simulink library "wt_blockset_v3"  (Simulink 6.0)
settings: Solver=ode45  SolverMode=SingleTasking  StartTime=0.0  StopTime=10.0  RelTol=1e-3
undefined symbols (not defined in the file): f1, get, j, Kmode, Type, u0
libraries: simulink_extras x12, simulink3 x5, simulink x4, dspinverses x1, dspmtrx3 x1, dspsnks4 x1
(part 3 of 7)

== system wt_blockset_v3/Mechanical Components/Wind Model SB-1 ==
  omg_wt : Inport  Port=1  LatchInput=off
  0 Harmonic Filter : TransferFcn  Numerator=[0 4.7869*d 0.9904]  Denominator=[7.6823*d^2 7.3518*d 1]
  3 Harmonic : Sum  SaturateOnIntegerOverflow=on  InputSameDT=on
  3 Harmonic Filter_1 : TransferFcn  Numerator=[0 0.2766*d 0.0307]  Denominator=[0.3691*d^2 1.7722*d 1]
  3 Harmonic Filter_2 : TransferFcn  Numerator=[0 0.2766*d 0.0307]  Denominator=[0.3691*d^2 1.7722*d 1]
  Clock : Clock
  Constant1 : Constant  Value=v_mean
  Gain : Gain  Gain=2*pi/60  SaturateOnIntegerOverflow=on
  Kaimal_Filter_1 : Subsystem
  Kaimal_Filter_2 : Subsystem
  Kaimal_Filter_3 : Subsystem
  Mux : Mux  Inputs=2
  Product : Product  SaturateOnIntegerOverflow=on  InputSameDT=on
  Product1 : Product  SaturateOnIntegerOverflow=on  InputSameDT=on
  Sum : Sum  SaturateOnIntegerOverflow=on  InputSameDT=on
  Sum2 : Sum  SaturateOnIntegerOverflow=on  InputSameDT=on
  Unit Delay : UnitDelay  SampleTime=T_sample
  Unit Delay1 : UnitDelay  SampleTime=T_sample
  White Noise_1 : Subsystem  mask(Continuous White Noise.){Cov=[1], Ts=T_sample, seed=[random(1)]}
      mask prompts: Cov "Noise Power:"; Ts "Sample Time:"
      mask help:
      | White noise for continuous (s-domain) systems.
      | Band-limited using zero-order-hold.
      mask init:
      | r = rand(1,12); r2 = [r(1),r;r,r(12)]; t =[1:13;1:13];
      mask Help: Implemented using white noise into Zero-Order Hold block. The seed and power can be vectors of the same length to produce a vector of white noise sources. For faster simulation, set sample time to the highest value possible but in accordance with the fastest dynamics of system.
      mask Display: plot(t(:),r2(:))
  White Noise_2 : Subsystem  mask(Continuous White Noise.){@1=[1], @2=T_sample, @3=[random(2)]}
      mask prompts: @1 "Noise Power:"; @2 "Sample Time:"; @3 "Seed"
      mask help:
      | White noise for continuous (s-domain) systems.
      | Band-limited using zero-order-hold.
      mask init:
      | Cov = @1; Ts = @2; seed = @3; r = rand(1,12); r2 = [r(1),r;r,r(12)]; t =[1:13;1:13];
      mask Help: Implemented using white noise into Zero-Order Hold block. The seed and power can be vectors of the same length to produce a vector of white noise sources. For faster simulation, set sample time to the highest value possible but in accordance with the fastest dynamics of system.
      mask Display: plot(t(:),r2(:))
  White Noise_3 : Subsystem  mask(Continuous White Noise.){@1=[1], @2=T_sample, @3=[random(3)]}
      mask prompts: @1 "Noise Power:"; @2 "Sample Time:"; @3 "Seed"
      mask help:
      | White noise for continuous (s-domain) systems.
      | Band-limited using zero-order-hold.
      mask init:
      | Cov = @1; Ts = @2; seed = @3; r = rand(1,12); r2 = [r(1),r;r,r(12)]; t =[1:13;1:13];
      mask Help: Implemented using white noise into Zero-Order Hold block. The seed and power can be vectors of the same length to produce a vector of white noise sources. For faster simulation, set sample time to the highest value possible but in accordance with the fastest dynamics of system.
      mask Display: plot(t(:),r2(:))
  cos fun : Fcn  Expr=sqrt(2)*cos(3*u[1]*u[2])
  sin fun : Fcn  Expr=sqrt(2)*sin(3*u[1]*u[2])
  wind : Outport  InitialOutput=[u0]
  wires:
  Kaimal_Filter_2/1(out_1) -> 3 Harmonic Filter_1/1
  Kaimal_Filter_3/1(out_1) -> 3 Harmonic Filter_2/1
  cos fun/1 -> Unit Delay/1
  sin fun/1 -> Unit Delay1/1
  Product/1 -> 3 Harmonic/1
  Product1/1 -> 3 Harmonic/2
  3 Harmonic Filter_2/1 -> Product1/2
  3 Harmonic/1 -> Sum/2
  0 Harmonic Filter/1 -> Sum2/2
  Sum2/1 -> Sum/1
  Constant1/1 -> Sum2/1
  Sum/1 -> wind/1
  Kaimal_Filter_1/1(out_1) -> 0 Harmonic Filter/1
  White Noise_1/1(Out_1) -> Kaimal_Filter_1/1(in_1)
  White Noise_2/1(Out_1) -> Kaimal_Filter_2/1(in_1)
  White Noise_3/1(Out_1) -> Kaimal_Filter_3/1(in_1)
  3 Harmonic Filter_1/1 -> Product/1
  Mux/1 -> cos fun/1, sin fun/1
  omg_wt/1 -> Gain/1
  Gain/1 -> Mux/1
  Unit Delay/1 -> Product/2
  Unit Delay1/1 -> Product1/1
  Clock/1 -> Mux/2

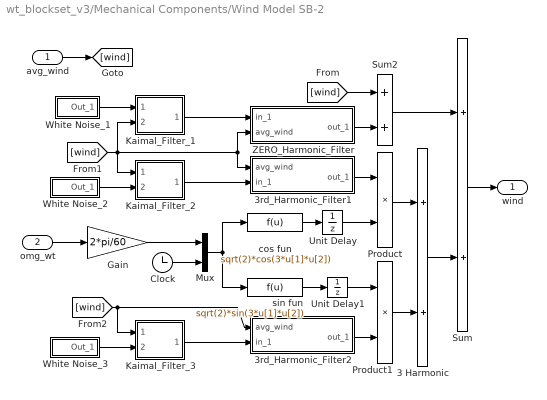
== system wt_blockset_v3/Mechanical Components/Wind Model SB-2 ==
  avg_wind : Inport  Port=1  LatchInput=off
  omg_wt : Inport  Port=2  LatchInput=off
  3 Harmonic : Sum  SaturateOnIntegerOverflow=on  InputSameDT=on
  3rd_Harmonic_Filter1 : Subsystem
  3rd_Harmonic_Filter2 : Subsystem
  Clock : Clock
  Gain : Gain  Gain=2*pi/60  SaturateOnIntegerOverflow=on
  Kaimal_Filter_1 : Subsystem
  Kaimal_Filter_2 : Subsystem
  Kaimal_Filter_3 : Subsystem
  Mux : Mux  Inputs=2
  Product : Product  SaturateOnIntegerOverflow=on  InputSameDT=on
  Product1 : Product  SaturateOnIntegerOverflow=on  InputSameDT=on
  Sum : Sum  SaturateOnIntegerOverflow=on  InputSameDT=on
  Sum2 : Sum  SaturateOnIntegerOverflow=on  InputSameDT=on
  Unit Delay : UnitDelay  SampleTime=T_sample
  Unit Delay1 : UnitDelay  SampleTime=T_sample
  White Noise_1 : Subsystem  mask(Continuous White Noise.){Cov=[1], Ts=T_sample, seed=[random(1)]}
      mask prompts: Cov "Noise Power:"; Ts "Sample Time:"
      mask help:
      | White noise for continuous (s-domain) systems.
      | Band-limited using zero-order-hold.
      mask init:
      | r = rand(1,12); r2 = [r(1),r;r,r(12)]; t =[1:13;1:13];
      mask Help: Implemented using white noise into Zero-Order Hold block. The seed and power can be vectors of the same length to produce a vector of white noise sources. For faster simulation, set sample time to the highest value possible but in accordance with the fastest dynamics of system.
      mask Display: plot(t(:),r2(:))
  White Noise_2 : Subsystem  mask(Continuous White Noise.){@1=[1], @2=T_sample, @3=[random(2)]}
      mask prompts: @1 "Noise Power:"; @2 "Sample Time:"; @3 "Seed"
      mask help:
      | White noise for continuous (s-domain) systems.
      | Band-limited using zero-order-hold.
      mask init:
      | Cov = @1; Ts = @2; seed = @3; r = rand(1,12); r2 = [r(1),r;r,r(12)]; t =[1:13;1:13];
      mask Help: Implemented using white noise into Zero-Order Hold block. The seed and power can be vectors of the same length to produce a vector of white noise sources. For faster simulation, set sample time to the highest value possible but in accordance with the fastest dynamics of system.
      mask Display: plot(t(:),r2(:))
  White Noise_3 : Subsystem  mask(Continuous White Noise.){@1=[1], @2=T_sample, @3=[random(3)]}
      mask prompts: @1 "Noise Power:"; @2 "Sample Time:"; @3 "Seed"
      mask help:
      | White noise for continuous (s-domain) systems.
      | Band-limited using zero-order-hold.
      mask init:
      | Cov = @1; Ts = @2; seed = @3; r = rand(1,12); r2 = [r(1),r;r,r(12)]; t =[1:13;1:13];
      mask Help: Implemented using white noise into Zero-Order Hold block. The seed and power can be vectors of the same length to produce a vector of white noise sources. For faster simulation, set sample time to the highest value possible but in accordance with the fastest dynamics of system.
      mask Display: plot(t(:),r2(:))
  ZERO_Harmonic_Filter : Subsystem
  cos fun : Fcn  Expr=sqrt(2)*cos(3*u[1]*u[2])
  sin fun : Fcn  Expr=sqrt(2)*sin(3*u[1]*u[2])
  wind : Outport  InitialOutput=[u0]
  wires:
  Clock/1 -> Mux/2
  Unit Delay1/1 -> Product1/1
  Unit Delay/1 -> Product/2
  Gain/1 -> Mux/1
  omg_wt/1 -> Gain/1
  Mux/1 -> sin fun/1, cos fun/1
  3rd_Harmonic_Filter1/1(out_1) -> Product/1
  White Noise_3/1(Out_1) -> Kaimal_Filter_3/2(in_1)
  White Noise_1/1(Out_1) -> Kaimal_Filter_1/1(in_1)
  Sum/1 -> wind/1
  [wind] -> Sum2/1
  Sum2/1 -> Sum/1
  ZERO_Harmonic_Filter/1(out_1) -> Sum2/2
  3 Harmonic/1 -> Sum/2
  3rd_Harmonic_Filter2/1(out_1) -> Product1/2
  Product1/1 -> 3 Harmonic/2
  Product/1 -> 3 Harmonic/1
  sin fun/1 -> Unit Delay1/1
  cos fun/1 -> Unit Delay/1
  Kaimal_Filter_1/1(out_1) -> ZERO_Harmonic_Filter/1(in_1)
  Kaimal_Filter_2/1(out_1) -> 3rd_Harmonic_Filter1/2(in_1)
  White Noise_2/1(Out_1) -> Kaimal_Filter_2/2(in_1)
  avg_wind/1 -> [wind]
  [wind] -> Kaimal_Filter_1/2(avg_wind), Kaimal_Filter_2/1(avg_wind), ZERO_Harmonic_Filter/2(avg_wind), 3rd_Harmonic_Filter1/1(avg_wind)
  [wind] -> Kaimal_Filter_3/1(avg_wind), 3rd_Harmonic_Filter2/1(avg_wind)
  Kaimal_Filter_3/1(out_1) -> 3rd_Harmonic_Filter2/2(in_1)

== system wt_blockset_v3/Mechanical Components/Wind Model ZA-1 ==
  omg_wt : Inport  Port=1  LatchInput=off
  0 Harmonic Filter : TransferFcn  Numerator=[0 4.7869*d 0.9904]  Denominator=[7.6823*d^2 7.3518*d 1]
  3 Harmonic : Sum  SaturateOnIntegerOverflow=on  InputSameDT=on
  3 Harmonic Filter_1 : TransferFcn  Numerator=[0 0.2766*d 0.0307]  Denominator=[0.3691*d^2 1.7722*d 1]
  3 Harmonic Filter_2 : TransferFcn  Numerator=[0 0.2766*d 0.0307]  Denominator=[0.3691*d^2 1.7722*d 1]
  Band Limited White Noise : Subsystem  mask(Band Limited White Noise Generator){noise=1, seed=256, T_sample=0.05}
      mask prompts: noise "noise power"; T_sample "sample time [sec]"
      mask help: Implements a Band Limited White Noise Generator using the Marsaglia's ziggurat method.
      mask Display: disp('White Noise')
  Band Limited White Noise1 : Subsystem  mask(Band Limited White Noise Generator){noise=1, seed=894, T_sample=0.05}
      mask prompts: noise "noise power"; T_sample "sample time [sec]"
      mask help: Implements a Band Limited White Noise Generator using the Marsaglia's ziggurat method.
      mask Display: disp('White Noise')
  Band Limited White Noise2 : Subsystem  mask(Band Limited White Noise Generator){noise=1, seed=31, T_sample=0.05}
      mask prompts: noise "noise power"; T_sample "sample time [sec]"
      mask help: Implements a Band Limited White Noise Generator using the Marsaglia's ziggurat method.
      mask Display: disp('White Noise')
  Clock : Clock
  Constant1 : Constant  Value=v_mean
  Gain : Gain  Gain=2*pi/60  SaturateOnIntegerOverflow=on
  Kaimal_Filter_1 : Subsystem
  Kaimal_Filter_2 : Subsystem
  Kaimal_Filter_3 : Subsystem
  Mux : Mux  Inputs=2
  Product : Product  SaturateOnIntegerOverflow=on  InputSameDT=on
  Product1 : Product  SaturateOnIntegerOverflow=on  InputSameDT=on
  Sum : Sum  SaturateOnIntegerOverflow=on  InputSameDT=on
  Sum2 : Sum  SaturateOnIntegerOverflow=on  InputSameDT=on
  Unit Delay2 : UnitDelay  SampleTime=T_sample
  Unit Delay3 : UnitDelay  SampleTime=T_sample
  cos fun : Fcn  Expr=sqrt(2)*cos(3*u[1]*u[2])
  sin fun : Fcn  Expr=sqrt(2)*sin(3*u[1]*u[2])
  wind : Outport  InitialOutput=[u0]
  wires:
  Band Limited White Noise2/1(wn) -> Kaimal_Filter_3/1(in_1)
  Band Limited White Noise1/1(wn) -> Kaimal_Filter_2/1(in_1)
  Band Limited White Noise/1(wn) -> Kaimal_Filter_1/1(in_1)
  Kaimal_Filter_1/1(out_1) -> 0 Harmonic Filter/1
  Sum/1 -> wind/1
  Constant1/1 -> Sum2/1
  Sum2/1 -> Sum/1
  0 Harmonic Filter/1 -> Sum2/2
  3 Harmonic/1 -> Sum/2
  3 Harmonic Filter_2/1 -> Product1/2
  Product/1 -> 3 Harmonic/1
  Kaimal_Filter_3/1(out_1) -> 3 Harmonic Filter_2/1
  Kaimal_Filter_2/1(out_1) -> 3 Harmonic Filter_1/1
  cos fun/1 -> Unit Delay2/1
  sin fun/1 -> Unit Delay3/1
  Mux/1 -> cos fun/1, sin fun/1
  omg_wt/1 -> Gain/1
  Gain/1 -> Mux/1
  Unit Delay2/1 -> Product/2
  Unit Delay3/1 -> Product1/1
  Clock/1 -> Mux/2
  3 Harmonic Filter_1/1 -> Product/1
  Product1/1 -> 3 Harmonic/2

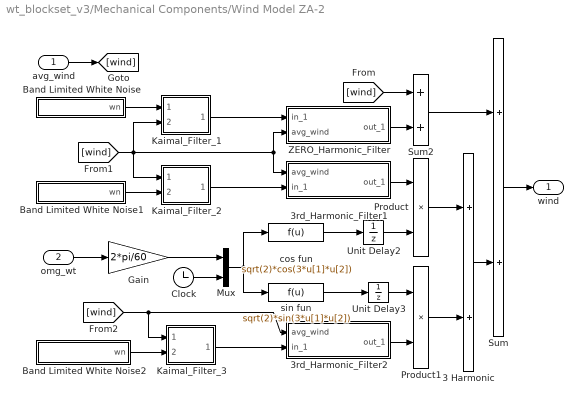
== system wt_blockset_v3/Mechanical Components/Wind Model ZA-2 ==
  avg_wind : Inport  Port=1  LatchInput=off
  omg_wt : Inport  Port=2  LatchInput=off
  3 Harmonic : Sum  SaturateOnIntegerOverflow=on  InputSameDT=on
  3rd_Harmonic_Filter1 : Subsystem
  3rd_Harmonic_Filter2 : Subsystem
  Band Limited White Noise : Subsystem  mask(Band Limited White Noise Generator){noise=1, seed=256, T_sample=0.05}
      mask prompts: noise "noise power"; T_sample "sample time [sec]"
      mask help: Implements a Band Limited White Noise Generator using the Marsaglia's ziggurat method.
      mask Display: disp('White Noise')
  Band Limited White Noise1 : Subsystem  mask(Band Limited White Noise Generator){noise=1, seed=894, T_sample=0.05}
      mask prompts: noise "noise power"; T_sample "sample time [sec]"
      mask help: Implements a Band Limited White Noise Generator using the Marsaglia's ziggurat method.
      mask Display: disp('White Noise')
  Band Limited White Noise2 : Subsystem  mask(Band Limited White Noise Generator){noise=1, seed=31, T_sample=0.05}
      mask prompts: noise "noise power"; T_sample "sample time [sec]"
      mask help: Implements a Band Limited White Noise Generator using the Marsaglia's ziggurat method.
      mask Display: disp('White Noise')
  Clock : Clock
  Gain : Gain  Gain=2*pi/60  SaturateOnIntegerOverflow=on
  Kaimal_Filter_1 : Subsystem
  Kaimal_Filter_2 : Subsystem
  Kaimal_Filter_3 : Subsystem
  Mux : Mux  Inputs=2
  Product : Product  SaturateOnIntegerOverflow=on  InputSameDT=on
  Product1 : Product  SaturateOnIntegerOverflow=on  InputSameDT=on
  Sum : Sum  SaturateOnIntegerOverflow=on  InputSameDT=on
  Sum2 : Sum  SaturateOnIntegerOverflow=on  InputSameDT=on
  Unit Delay2 : UnitDelay  SampleTime=T_sample
  Unit Delay3 : UnitDelay  SampleTime=T_sample
  ZERO_Harmonic_Filter : Subsystem
  cos fun : Fcn  Expr=sqrt(2)*cos(3*u[1]*u[2])
  sin fun : Fcn  Expr=sqrt(2)*sin(3*u[1]*u[2])
  wind : Outport  InitialOutput=[u0]
  wires:
  [wind] -> Kaimal_Filter_3/1(avg_wind), 3rd_Harmonic_Filter2/1(avg_wind)
  [wind] -> 3rd_Harmonic_Filter1/1(avg_wind), ZERO_Harmonic_Filter/2(avg_wind), Kaimal_Filter_2/1(avg_wind), Kaimal_Filter_1/2(avg_wind)
  Band Limited White Noise1/1(wn) -> Kaimal_Filter_2/2(in_1)
  Kaimal_Filter_2/1(out_1) -> 3rd_Harmonic_Filter1/2(in_1)
  Kaimal_Filter_1/1(out_1) -> ZERO_Harmonic_Filter/1(in_1)
  Band Limited White Noise/1(wn) -> Kaimal_Filter_1/1(in_1)
  [wind] -> Sum2/1
  avg_wind/1 -> [wind]
  Kaimal_Filter_3/1(out_1) -> 3rd_Harmonic_Filter2/2(in_1)
  Band Limited White Noise2/1(wn) -> Kaimal_Filter_3/2(in_1)
  Sum/1 -> wind/1
  Sum2/1 -> Sum/1
  ZERO_Harmonic_Filter/1(out_1) -> Sum2/2
  3 Harmonic/1 -> Sum/2
  3rd_Harmonic_Filter2/1(out_1) -> Product1/2
  Product/1 -> 3 Harmonic/1
  cos fun/1 -> Unit Delay2/1
  sin fun/1 -> Unit Delay3/1
  Mux/1 -> cos fun/1, sin fun/1
  omg_wt/1 -> Gain/1
  Gain/1 -> Mux/1
  Unit Delay2/1 -> Product/2
  Unit Delay3/1 -> Product1/1
  Clock/1 -> Mux/2
  3rd_Harmonic_Filter1/1(out_1) -> Product/1
  Product1/1 -> 3 Harmonic/2

== system wt_blockset_v3/Mechanical Components/Wind Turbine Rotor Active Stall ==
  pitch : Inport  Port=1  LatchInput=off
  wind : Inport  Port=2  LatchInput=off
  omg_wt : Inport  Port=3  LatchInput=off
  Actuator : TransferFcn  Denominator=[Tact 1]
  Cq  look-up table : S-Function  FunctionName=sfun_lookupnd  Parameters=numDims,tableData,bp1,bp2,bp3,bp4,bpcell,searchMode,cacheBpFlag,vectorInputFlag,interpMethod,extrapMethod,rangeErrorMode  mask(LookupNDInterp){numDimsPopupSelect=2, bp1=[0:1:20], bp2=[-90:5:90], bp3=[1:3], bp4=[1:3], bpcell={ [1:3], [1:3] }, explicitNumDims=2, searchMode=Binary Search, cacheBpFlag=off, vectorInputFlag=off, tableData=Ctorque, interpMethod=Linear, extrapMethod=None - Clip, rangeErrorMode=Error}
      mask prompts: numDimsPopupSelect "Number of table dimensions:"; bp1 "First input (row) breakpoint set:"; bp2 "Second (column) input breakpoint set:"; bp3 "Third input breakpoint set:"; bp4 "Fourth input breakpoint set:"; bpcell "Fifth..Nth breakpoint sets (cell array):"; explicitNumDims "Explicit number of dimensions:"; searchMode "Index search method:"; cacheBpFlag "Begin index searches using previous index results"; vectorInputFlag "Use one (vector) input port instead of N ports"; tableData "Table data:"; interpMethod "Interpolation method:"; extrapMethod "Extrapolation method:"; rangeErrorMode "Action for out of range input:"
      mask help: Perform n-dimensional interpolated table lookup including index searches. The table is a sampled representation of a function in N variables. Breakpoint sets relate the input values to positions in the table. The first dimension corresponds to the top (or left) input port.
      mask init:
      | if numDimsPopupSelect==5
      |   numDims=explicitNumDims;
      | else
      |   numDims=numDimsPopupSelect;
      | end
      | if strcmp(get_param(bdroot,'BlockDiagramType'),'library')
      |   dimsChar = 'n';
      | else
      |   dimsChar = sprintf('%d',numDims);
      | end
      | switch interpMethod
      |   case 1
      |     plottype = 'flatplot';
      |   case 2
      |     plottype = 'lineplot';
      |   otherwise
      |     plottype = 'splineplot';
      | end
      | 
      | [x,y,xaxes,yaxes] = ndlookico(plottype, numDims, 'LookupNDInterp', tableData, bp1);
      mask StyleString: popup(   1   |   2   |   3   |   4   |More...),edit,edit,edit,edit,edit,edit,popup(Evenly Spaced Points|Linear Search|Binary Search),checkbox,checkbox,edit,popup(None - Flat|Linear|Cubic Spline),popup(None - Clip|Linear|Cubic Spline),popup(None|Warning|Error)
      mask CallbackString: ndlookico|||||||||||||
      mask Display:
      | text(0.5,0.9,sprintf(' %s-D T(u)',dimsChar),'horizontalAlignment','center')
      | plot(x,y)
      | plot(xaxes,yaxes)
  Logical Operator : Logic
  Mux : Mux  Inputs=2
  Mux1 : Mux  Inputs=2
  Relational Operator : RelationalOperator  InputSameDT=on
  Relational Operator1 : RelationalOperator  Operator=<=  InputSameDT=on
  Saturation : Saturate  UpperLimit=20  LowerLimit=-20
  Switch : Switch  Threshold=.5  SaturateOnIntegerOverflow=on  InputSameDT=on
  Torque : Fcn  Expr=-0.5*pi*ro_air*(R^3)*(u(1)^2)*u(2)
  cut_in : Constant  Value=cut_in
  cut_out : Constant  Value=cut_out
  lamda : Fcn  Expr=u(2)*R/u(1)
  null : Constant  Value=0
  T_wt : Outport
  wires:
  Mux/1 -> lamda/1
  Mux1/1 -> Torque/1
  omg_wt/1 -> Mux/2
  cut_in/1 -> Relational Operator/2
  cut_out/1 -> Relational Operator1/2
  Relational Operator1/1 -> Logical Operator/2
  Relational Operator/1 -> Logical Operator/1
  Switch/1 -> T_wt/1
  Torque/1 -> Switch/1
  null/1 -> Switch/3
  Logical Operator/1 -> Switch/2
  wind/1 -> Mux/1, Relational Operator/1, Relational Operator1/1, Mux1/1
  Cq  look-up table/1 -> Mux1/2
  lamda/1 -> Cq  look-up table/1
  pitch/1 -> Saturation/1
  Saturation/1 -> Actuator/1
  Actuator/1 -> Cq  look-up table/2

== system wt_blockset_v3/Mechanical Components/Wind Turbine Rotor Variable Pitch ==
  pitch : Inport  Port=1  LatchInput=off
  wind : Inport  Port=2  LatchInput=off
  omg_wt : Inport  Port=3  LatchInput=off
  Actuator : TransferFcn  Denominator=[Tact 1]
  Cq  look-up table : S-Function  FunctionName=sfun_lookupnd  Parameters=numDims,tableData,bp1,bp2,bp3,bp4,bpcell,searchMode,cacheBpFlag,vectorInputFlag,interpMethod,extrapMethod,rangeErrorMode  mask(LookupNDInterp){numDimsPopupSelect=2, bp1=[0:1:20], bp2=[-90:5:90], bp3=[1:3], bp4=[1:3], bpcell={ [1:3], [1:3] }, explicitNumDims=2, searchMode=Binary Search, cacheBpFlag=off, vectorInputFlag=off, tableData=Ctorque, interpMethod=Linear, extrapMethod=None - Clip, rangeErrorMode=Error}
      mask prompts: numDimsPopupSelect "Number of table dimensions:"; bp1 "First input (row) breakpoint set:"; bp2 "Second (column) input breakpoint set:"; bp3 "Third input breakpoint set:"; bp4 "Fourth input breakpoint set:"; bpcell "Fifth..Nth breakpoint sets (cell array):"; explicitNumDims "Explicit number of dimensions:"; searchMode "Index search method:"; cacheBpFlag "Begin index searches using previous index results"; vectorInputFlag "Use one (vector) input port instead of N ports"; tableData "Table data:"; interpMethod "Interpolation method:"; extrapMethod "Extrapolation method:"; rangeErrorMode "Action for out of range input:"
      mask help: Perform n-dimensional interpolated table lookup including index searches. The table is a sampled representation of a function in N variables. Breakpoint sets relate the input values to positions in the table. The first dimension corresponds to the top (or left) input port.
      mask init: same as wt_blockset_v3/Mechanical Components/Wind Turbine Rotor Active Stall/Cq  look-up table
      mask StyleString: popup(   1   |   2   |   3   |   4   |More...),edit,edit,edit,edit,edit,edit,popup(Evenly Spaced Points|Linear Search|Binary Search),checkbox,checkbox,edit,popup(None - Flat|Linear|Cubic Spline),popup(None - Clip|Linear|Cubic Spline),popup(None|Warning|Error)
      mask CallbackString: ndlookico|||||||||||||
      mask Display:
      | text(0.5,0.9,sprintf(' %s-D T(u)',dimsChar),'horizontalAlignment','center')
      | plot(x,y)
      | plot(xaxes,yaxes)
  Logical Operator : Logic
  Mux : Mux  Inputs=2
  Mux1 : Mux  Inputs=2
  Relational Operator : RelationalOperator  InputSameDT=on
  Relational Operator1 : RelationalOperator  Operator=<=  InputSameDT=on
  Switch : Switch  Threshold=.5  SaturateOnIntegerOverflow=on  InputSameDT=on
  Torque : Fcn  Expr=-0.5*pi*ro_air*(R^3)*(u(1)^2)*u(2)
  cut_in : Constant  Value=cut_in
  cut_out : Constant  Value=cut_out
  lamda : Fcn  Expr=u(2)*R/u(1)
  null : Constant  Value=0
  T_wt : Outport
  wires:
  pitch/1 -> Actuator/1
  lamda/1 -> Cq  look-up table/1
  Cq  look-up table/1 -> Mux1/2
  wind/1 -> Mux1/1, Relational Operator1/1, Relational Operator/1, Mux/1
  Logical Operator/1 -> Switch/2
  null/1 -> Switch/3
  Torque/1 -> Switch/1
  Switch/1 -> T_wt/1
  Relational Operator/1 -> Logical Operator/1
  Relational Operator1/1 -> Logical Operator/2
  cut_out/1 -> Relational Operator1/2
  cut_in/1 -> Relational Operator/2
  omg_wt/1 -> Mux/2
  Mux1/1 -> Torque/1
  Mux/1 -> lamda/1
  Actuator/1 -> Cq  look-up table/2

== system wt_blockset_v3/Power Converters/3-phase Diode Bridge Rectifier ==
  note: Phase Voltage
  note: Phase Current
  note: DC-link Current
  v_ph : Inport  Port=1  LatchInput=off
  Idc : Inport  Port=2  LatchInput=off
  DC-link Voltage : Fcn  Expr=u(1)+u(2)+u(3)
  Diode  State Calculator : Subsystem
  Product1 : Product  SaturateOnIntegerOverflow=on  InputSameDT=on
  Product3 : Product  SaturateOnIntegerOverflow=on  InputSameDT=on
  i_ph : Outport  InitialOutput=0
  Vdc : Outport  Port=2  InitialOutput=0
  wires:
  v_ph/1 -> Diode  State Calculator/1(RST), Product3/1
  Product3/1 -> DC-link Voltage/1
  DC-link Voltage/1 -> Vdc/1
  Diode  State Calculator/1(K) -> Product3/2, Product1/1
  Idc/1 -> Product1/2
  Product1/1 -> i_ph/1

== system wt_blockset_v3/Power Converters/Average PWM Strategy ==
  vd_ref : Inport  Port=1  LatchInput=off
  vq_ref : Inport  Port=2  LatchInput=off
  Vdc : Inport  Port=3  LatchInput=off
  freq : Inport  Port=4  LatchInput=off
  Gain : Gain  Gain=2*pi  SaturateOnIntegerOverflow=on
  Integrator : Integrator
  Mux : Mux  Inputs=2
  Mux1 : Mux  Inputs=3
  Mux2 : Mux  Inputs=3
  duty_A1 : Fcn  Expr=0.5*2/sqrt(3)*u(1)*(sin(u(2))+(sin(3*u(2))/6)*(third==1))
  duty_A2 : Fcn  Expr=0.5*2/sqrt(3)*u(1)*(sin(u(2)-2*pi/3)+(sin(3*u(2))/6)*(third==1))
  duty_A3 : Fcn  Expr=0.5*2/sqrt(3)*u(1)*(sin(u(2)+2*pi/3)+(sin(3*u(2))/6)*(third==1))
  ma : Fcn  Expr=sqrt(3)/2*sqrt(u(1)^2+u(3)^2)/u(2)
  duty_ABC : Outport
  wires:
  freq/1 -> Gain/1
  Mux/1 -> duty_A1/1, duty_A2/1, duty_A3/1
  Integrator/1 -> Mux/2
  Gain/1 -> Integrator/1
  duty_A1/1 -> Mux1/1
  duty_A2/1 -> Mux1/2
  duty_A3/1 -> Mux1/3
  Mux2/1 -> ma/1
  ma/1 -> Mux/1
  vd_ref/1 -> Mux2/1  "vdref"
  Vdc/1 -> Mux2/2  "vdc"
  vq_ref/1 -> Mux2/3  "vqref"
  Mux1/1 -> duty_ABC/1

== system wt_blockset_v3/Power Converters/Average SVM Strategy ==
  vd_ref : Inport  Port=1  LatchInput=off
  vq_ref : Inport  Port=2  LatchInput=off
  Vdc : Inport  Port=3  LatchInput=off
  1st quadrant : Subsystem  TreatAsAtomicUnit=on
  2nd quadrant : Subsystem  TreatAsAtomicUnit=on
  3rd quadrant : Subsystem  TreatAsAtomicUnit=on
  4th quadrant : Subsystem  TreatAsAtomicUnit=on
  "Avoid saturation " : Subsystem
      mask Display: disp('Avoid\nSaturation')
  If : If  NumInputs=2  IfExpression=(u1 >= 0)&(u2 >=0)  ElseIfExpressions=(u1 < 0)&(u2 > 0), (u1 < 0)&(u2 <=0), (u1 >= 0)&(u2 <0)  ShowElse=off
  Sum : Sum  Inputs=++++  SaturateOnIntegerOverflow=on
  Weight : Subsystem
      mask Type: Avoid saturation
      mask Display: disp('Weight')
  capcom duty cycle : Subsystem
  duty_ABC : Outport
  tag scope: vdc=global, vdref=global, vqref=global
  wires:
  vd_ref/1 -> [vdref]  "vdref"
  vq_ref/1 -> [vqref]  "vqref"
  Vdc/1 -> [vdc]  "vdc"
  [vd] -> If/1
  [vq] -> If/2
  If/1 -> 1st quadrant/Action
  [vd] -> 1st quadrant/1(vd)
  [vq] -> 1st quadrant/2(vq)
  [vd] -> 2nd quadrant/1(vd)
  [vq] -> 2nd quadrant/2(vq)
  If/2 -> 2nd quadrant/Action
  [vd] -> 3rd quadrant/1(vd)
  [vq] -> 3rd quadrant/2(vq)
  If/3 -> 3rd quadrant/Action
  [vd] -> 4th quadrant/1(vd)
  [vq] -> 4th quadrant/2(vq)
  If/4 -> 4th quadrant/Action
  1st quadrant/1(duty_ABC) -> Sum/1
  2nd quadrant/1(duty_ABC) -> Sum/2
  4th quadrant/1(duty_ABC) -> Sum/4
  3rd quadrant/1(duty_ABC) -> Sum/3
  Sum/1 -> capcom duty cycle/1(duty_ABC)
  capcom duty cycle/1(pwm_abc) -> duty_ABC/1

== system wt_blockset_v3/Power Converters/Average SVM Strategy C_Sfun ==
  vd_ref : Inport  Port=1  LatchInput=off
  vq_ref : Inport  Port=2  LatchInput=off
  Vdc : Inport  Port=3  LatchInput=off
  Mux : Mux  Inputs=3
  SVM : S-Function  FunctionName=space_vector_mod_sat
  capcom duty cycle : Subsystem
  duty_ABC : Outport
  wires:
  capcom duty cycle/1(pwm_abc) -> duty_ABC/1
  Mux/1 -> SVM/1
  vd_ref/1 -> Mux/1
  vq_ref/1 -> Mux/2
  Vdc/1 -> Mux/3
  SVM/1 -> capcom duty cycle/1(duty_ABC)

== system wt_blockset_v3/Power Converters/RMS - Soft Starter ==
  phase : Inport  Port=1  LatchInput=off
  |V| : Inport  Port=2  LatchInput=off
  alpha : Inport  Port=3  LatchInput=off
  Look-up table extinction angle : Subsystem
  Mux : Mux  Inputs=3
  deg->rad : Gain  Gain=pi/180  SaturateOnIntegerOverflow=on
  deg->rad1 : Gain  Gain=pi/180  SaturateOnIntegerOverflow=on
  output voltage : Fcn  Expr=u(1)*sqrt((u(3)-u(2)+0.5*sin(2*u(2))-0.5*sin(2*u(3)))/pi)
  Vout : Outport
  wires:
  Look-up table extinction angle/1(extinction) -> deg->rad1/1
  deg->rad1/1 -> Mux/3
  deg->rad/1 -> Mux/2
  Mux/1 -> output voltage/1
  |V|/1 -> Mux/1
  output voltage/1 -> Vout/1
  alpha/1 -> Look-up table extinction angle/1(firing angle), deg->rad/1
  phase/1 -> Look-up table extinction angle/2(phase)

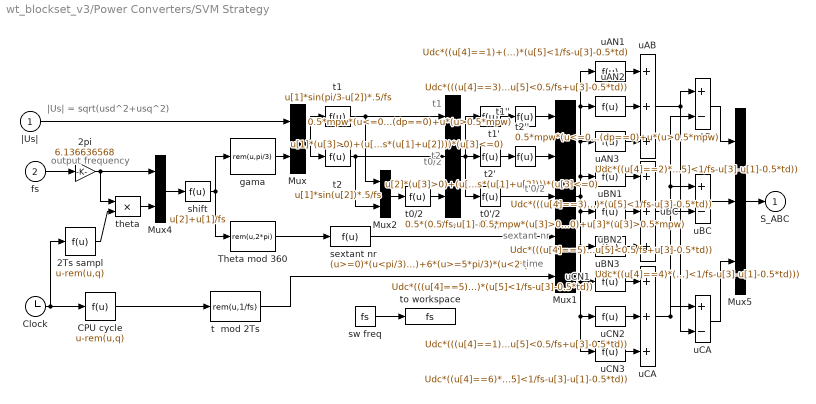
== system wt_blockset_v3/Power Converters/SVM Strategy ==
  note: |Us| = sqrt(usd^2+usq^2)
  note: output frequency
  note: t'0/2
  note: sextant nr
  note: t0/2
  note: t2
  note: t1
  note: time
  |Us| : Inport  Port=1  LatchInput=off
  fs : Inport  Port=2  LatchInput=off
  " sextant nr" : Fcn  Expr=(u>=0)*(u<pi/3)+2*(u>=pi/3)*(u<2*pi/3)+3*(u>=2*pi/3)*(u<pi)+4*(u>=pi)*(u<4*pi/3)+5*(u>=4*pi/3)*(u<5*pi/3)+6*(u>=5*pi/3)*(u<2*pi)
  " to workspace" : ToWorkspace  VariableName=fs  SaveFormat=Array
      settings: MaxDataPoints=1
  2Ts sampl : Fcn  Expr=u-rem(u,q)  mask(Quantizer){@1=1/fs}
      mask prompts: @1 "Quantization interval:"
      mask help: Discretizes input at given interval.
      mask init:
      | q = @1;
      mask Help: Quantizes input in given intervals.
      mask Display: plot([10,0],[5,5],[5,5],[0,10],[1,2,2,3,3,4,4,5,5,6,6,7,7,8,8,9,9],[1,1,2,2,3,3,4,4,5,5,6,6,7,7,8,8,9])
  2pi : Gain  Gain=6.136636568  SaturateOnIntegerOverflow=on
  CPU cycle : Fcn  Expr=u-rem(u,q)  mask(Quantizer){@1=mct}
      mask prompts: @1 "Quantization interval:"
      mask help: Discretizes input at given interval.
      mask init:
      | q = @1;
      mask Help: Quantizes input in given intervals.
      mask Display: plot([10,0],[5,5],[5,5],[0,10],[1,2,2,3,3,4,4,5,5,6,6,7,7,8,8,9,9],[1,1,2,2,3,3,4,4,5,5,6,6,7,7,8,8,9])
  Clock : Clock
      settings: Decimation=10
  Mux : Mux  Inputs=2
  Mux1 : Mux  Inputs=5
  Mux2 : Mux  Inputs=2
  Mux3 : Mux  Inputs=3
  Mux4 : Mux  Inputs=2
  Mux5 : Mux  Inputs=3
  Theta mod 360 : MATLABFcn  MATLABFcn=rem(u,2*pi)
  gama : MATLABFcn  MATLABFcn=rem(u,pi/3)
  shift : Fcn  Expr=u[2]+u[1]/fs
  sw freq : Constant  Value=fs
  t  mod 2Ts : MATLABFcn  MATLABFcn=rem(u,1/fs)
  t0'/2 : Fcn  Expr=0.5*mpw*(u[3]>0)*(u[3]<=0.5*mpw)*(dp==0)+u[3]*(u[3]>0.5*mpw)
  t0/2 : Fcn  Expr=0.5*(0.5/fs-u[1]-u[2])
  t1 : Fcn  Expr=u[1]*sin(pi/3-u[2])*.5/fs
  t1' : Fcn  Expr=u[1]*(u[3]>0)+(u[1]/(2*fs*(u[1]+u[2])))*(u[3]<=0)
  t1'' : Fcn  Expr=0.5*mpw*(u<=0.5*mpw)*(dp==0)+u*(u>0.5*mpw)
  t2 : Fcn  Expr=u[1]*sin(u[2])*.5/fs
  t2' : Fcn  Expr=u[2]*(u[3]>0)+(u[2]/(2*fs*(u[1]+u[2])))*(u[3]<=0)
  t2'' : Fcn  Expr=0.5*mpw*(u<=0.5*mpw)*(dp==0)+u*(u>0.5*mpw)
  theta : Product  SaturateOnIntegerOverflow=on  InputSameDT=on
  uAB : Sum  Inputs=+++  SaturateOnIntegerOverflow=on  InputSameDT=on
  "uAB  " : Sum  Inputs=+-  SaturateOnIntegerOverflow=on  InputSameDT=on
  uAN1 : Fcn  Expr=Udc*((u[4]==1)+(u[4]==6))*(u[5]>=u[3]+0.5*td)*(u[5]<1/fs-u[3]-0.5*td)
  uAN2 : Fcn  Expr=Udc*(((u[4]==3)+(u[4]==4))*(u[5]>=0.5/fs-u[3]+0.5*td)*(u[5]<0.5/fs+u[3]-0.5*td))
  uAN3 : Fcn  Expr=Udc*((u[4]==2)*(u[5]>=u[3]+u[2]+0.5*td)*(u[5]<1/fs-u[3]-u[2]-0.5*td)+(u[4]==5)*(u[5]>=u[3]+u[1]+0.5*td)*(u[5]<1/fs-u[3]-u[1]-0.5*td))
  uBC : Sum  Inputs=+++  SaturateOnIntegerOverflow=on  InputSameDT=on
  "uBC  " : Sum  Inputs=+-  SaturateOnIntegerOverflow=on  InputSameDT=on
  uBN1 : Fcn  Expr=Udc*(((u[4]==3)+(u[4]==2))*(u[5]>=u[3]+0.5*td)*(u[5]<1/fs-u[3]-0.5*td))
  uBN2 : Fcn  Expr=Udc*(((u[4]==5)+(u[4]==6))*(u[5]>=0.5/fs-u[3]+0.5*td)*(u[5]<0.5/fs+u[3]-0.5*td))
  uBN3 : Fcn  Expr=Udc*((u[4]==4)*((u[5]>=u[3]+u[2]+0.5*td)*(u[5]<1/fs-u[3]-u[2]-0.5*td))+(u[4]==1)*((u[5]>=u[3]+u[1]+0.5*td)*(u[5]<1/fs-u[3]-u[1]-0.5*td)))
  uCA : Sum  Inputs=+++  SaturateOnIntegerOverflow=on  InputSameDT=on
  "uCA  " : Sum  Inputs=+-  SaturateOnIntegerOverflow=on  InputSameDT=on
  uCN1 : Fcn  Expr=Udc*(((u[4]==5)+(u[4]==4))*(u[5]>=u[3]+0.5*td)*(u[5]<1/fs-u[3]-0.5*td))
  uCN2 : Fcn  Expr=Udc*(((u[4]==1)+(u[4]==2))*(u[5]>=0.5/fs-u[3]+0.5*td)*(u[5]<0.5/fs+u[3]-0.5*td))
  uCN3 : Fcn  Expr=Udc*((u[4]==6)*(u[5]>=u[3]+u[2]+0.5*td)*(u[5]<1/fs-u[3]-u[2]-0.5*td)+(u[4]==3)*(u[5]>=u[3]+u[1]+0.5*td)*(u[5]<1/fs-u[3]-u[1]-0.5*td))
  S_ABC : Outport
  wires:
  sw freq/1 -> " to workspace"/1
  uAB/1 -> "uCA  "/2, "uAB  "/1
  |Us|/1 -> Mux/1
  fs/1 -> 2pi/1
  Mux4/1 -> shift/1
  theta/1 -> Mux4/2
  uCA/1 -> "uBC  "/2, "uCA  "/1
  uBC/1 -> "uAB  "/2, "uBC  "/1
  t2''/1 -> Mux1/2
  t1''/1 -> Mux1/1
  t1'/1 -> t1''/1
  t0'/2/1 -> Mux1/3
  t2'/1 -> t2''/1
  Mux3/1 -> t1'/1, t0'/2/1, t2'/1
  CPU cycle/1 -> t  mod 2Ts/1
  Clock/1 -> 2Ts sampl/1, CPU cycle/1
  Theta mod 360/1 -> " sextant nr"/1
  gama/1 -> Mux/2
  Mux2/1 -> t0/2/1
  uBN1/1 -> uBC/1
  uBN2/1 -> uBC/2
  uCN1/1 -> uCA/1
  uCN2/1 -> uCA/2
  " sextant nr"/1 -> Mux1/4
  Mux/1 -> t2/1, t1/1
  t2/1 -> Mux2/2, Mux3/2
  t0/2/1 -> Mux3/3
  2pi/1 -> Mux4/1, theta/1
  2Ts sampl/1 -> theta/2
  shift/1 -> gama/1, Theta mod 360/1
  t  mod 2Ts/1 -> Mux1/5
  uCN3/1 -> uCA/3
  uBN3/1 -> uBC/3
  uAN3/1 -> uAB/3
  uAN1/1 -> uAB/1
  uAN2/1 -> uAB/2
  Mux1/1 -> uAN1/1, uAN2/1, uAN3/1, uBN1/1, uBN2/1, uBN3/1, uCN1/1, uCN3/1, uCN2/1
  t1/1 -> Mux3/1, Mux2/1
  "uAB  "/1 -> Mux5/1
  "uBC  "/1 -> Mux5/2
  "uCA  "/1 -> Mux5/3
  Mux5/1 -> S_ABC/1

== system wt_blockset_v3/Power Converters/Sinus PWM ==
  Uabc_ref : Inport  Port=1  LatchInput=off
  Mux : Mux  Inputs=3
  Reshape : S-Function  FunctionName=sreshape  Parameters=OutputDimensionality, OutputDimensions  mask(Reshape){OutputDimensionality=1-D array, OutputDimensions=[1,1]}
      mask prompts: OutputDimensionality "Output dimensionality:"; OutputDimensions "Output dimensions:"
      mask help:
      | Change the dimensions of a vector or matrix input signal. Output
      |  - a one-dimensional array (vector),
      |  - a column vector (Mx1 matrix),
      |  - a row vector (1xN matrix), or
      |  - a matrix or vector with specified dimensions, e.g., [M, N] or [W].
      mask init:
      | s = reshapemask(gcb,'init');
      mask StyleString: popup(1-D array|Column vector|Row vector|Customize),edit
      mask CallbackString: reshapemask(gcb,'cbDimensionality')|
      mask Display: disp('U( : )')
  Selector : Selector  Elements=[1]  InputPortWidth=3
  Selector1 : Selector  Elements=[1]  InputPortWidth=3
  Sum : Sum  Inputs=-+  SaturateOnIntegerOverflow=on  InputSameDT=on
  Vtri : Subsystem  mask{fsw=mf*f1}
      mask prompts: fsw "switching frequency"
      mask init:
      | fsw2=fsw*2;
      | x=[0 1/4 3/4 1];
      | y=[0 -1     1    0];
      mask Display: plot([x  x+1 ],[y y])
  logical : Subsystem
      mask init:
      | x=[-5 0 0 5];
      | y=[ 0 0 1 1];
      mask Display: plot(x,y)
  test : Scope
      settings: TickLabels=on  TimeRange=0.02  YMin=-1.1  YMax=1.1
  S_ABC : Outport
  wires:
  logical/1(Out1) -> Reshape/1  "q"
  Vtri/1(Vtri) -> Sum/1, Mux/3  "Vtri"
  Uabc_ref/1 -> Sum/2, Selector/1  "Vcontrol"
  Sum/1 -> logical/1(In1)
  Selector1/1 -> Mux/1
  Selector/1 -> Mux/2
  Mux/1 -> test/1
  Reshape/1 -> S_ABC/1, Selector1/1  "q"

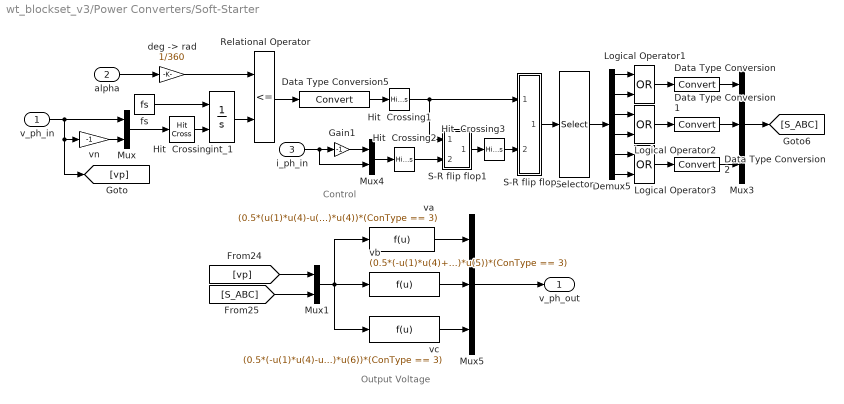
== system wt_blockset_v3/Power Converters/Soft-Starter ==
  note: Output Voltage
  note: Control
  v_ph_in : Inport  Port=1  LatchInput=off
  alpha : Inport  Port=2  LatchInput=off
  i_ph_in : Inport  Port=3  LatchInput=off
  Data Type Conversion{,1..2,5} (4 alike) : DataTypeConversion  OutDataTypeMode=double  SaturateOnIntegerOverflow=on  RndMeth=Zero
  Demux5 : Demux  Outputs=6
  Gain1 : Gain  Gain=-1  SaturateOnIntegerOverflow=on
  Hit  Crossing : HitCross  HitCrossingDirection=rising
  Hit  Crossing1 : HitCross  HitCrossingDirection=rising
  Hit  Crossing2 : HitCross  HitCrossingOffset=1  HitCrossingDirection=falling
  Hit  Crossing3 : HitCross  HitCrossingDirection=rising
  Logical Operator1 : Logic  Operator=OR
  Logical Operator2 : Logic  Operator=OR
  Logical Operator3 : Logic  Operator=OR
  Mux : Mux  Inputs=2
  Mux1 : Mux  Inputs=[3 3]
  Mux3 : Mux  Inputs=3
  Mux4 : Mux  Inputs=2
  Mux5 : Mux  Inputs=3
  Relational Operator : RelationalOperator  Operator=<=  InputSameDT=on
  S-R flip flop : Subsystem
  S-R flip flop1 : Subsystem
  Selector : Selector  Elements=[1 4 2 5 3 6]  InputPortWidth=6
  "deg -> rad" : Gain  Gain=1/360  SaturateOnIntegerOverflow=on
  fs : Constant  Value=fs
  int_1 : Integrator  ExternalReset=falling
  va : Fcn  Expr=(0.5*(u(1)*u(4)-u(2)*u(5)-u(3)*u(6)))*(ConType == 1)+(u(1)*(u(4)*(u(5))))*(ConType == 2)+(u(1)*u(4))*(ConType == 3)
  vb : Fcn  Expr=(0.5*(-u(1)*u(4)+u(2)*u(5)-u(3)*u(6)))*(ConType == 1)+(u(2)*(u(5)*(u(6))))*(ConType == 2)+(u(2)*u(5))*(ConType == 3)
  vc : Fcn  Expr=(0.5*(-u(1)*u(4)-u(2)*u(5)+u(3)*u(6)))*(ConType == 1)+(u(3)*(u(6)*(u(4))))*(ConType == 2)+(u(3)*u(6))*(ConType == 3)
  vn : Gain  Gain=-1  SaturateOnIntegerOverflow=on
  v_ph_out : Outport
  wires:
  S-R flip flop1/1(Q) -> Hit  Crossing3/1
  Hit  Crossing3/1 -> S-R flip flop/2(R)
  Gain1/1 -> Mux4/1
  Hit  Crossing2/1 -> S-R flip flop1/2(S)
  Mux4/1 -> Hit  Crossing2/1
  Data Type Conversion2/1 -> Mux3/3
  Data Type Conversion1/1 -> Mux3/2
  vc/1 -> Mux5/3
  vb/1 -> Mux5/2
  va/1 -> Mux5/1
  Mux5/1 -> v_ph_out/1
  [S_ABC] -> Mux1/2
  [vp] -> Mux1/1
  Mux3/1 -> [S_ABC]
  Data Type Conversion/1 -> Mux3/1
  Mux1/1 -> vc/1, vb/1, va/1
  Hit  Crossing/1 -> int_1/2
  fs/1 -> int_1/1
  Relational Operator/1 -> Data Type Conversion5/1
  int_1/1 -> Relational Operator/2
  "deg -> rad"/1 -> Relational Operator/1
  alpha/1 -> "deg -> rad"/1
  S-R flip flop/1(Q) -> Selector/1
  Mux/1 -> Hit  Crossing/1
  v_ph_in/1 -> [vp], vn/1, Mux/1
  vn/1 -> Mux/2
  Demux5/1 -> Logical Operator1/1
  Demux5/2 -> Logical Operator1/2
  Demux5/3 -> Logical Operator2/1
  Demux5/4 -> Logical Operator2/2
  Demux5/5 -> Logical Operator3/1
  Demux5/6 -> Logical Operator3/2
  Logical Operator1/1 -> Data Type Conversion/1
  Logical Operator2/1 -> Data Type Conversion1/1
  Logical Operator3/1 -> Data Type Conversion2/1
  Selector/1 -> Demux5/1
  Hit  Crossing1/1 -> S-R flip flop/1(S), S-R flip flop1/1(R)
  Data Type Conversion5/1 -> Hit  Crossing1/1
  i_ph_in/1 -> Mux4/2, Gain1/1

== system wt_blockset_v3/Power Converters/Switching PWM Strategy ==
  vd_ref : Inport  Port=1  LatchInput=off
  vq_ref : Inport  Port=2  LatchInput=off
  Vdc : Inport  Port=3  LatchInput=off
  freq : Inport  Port=4  LatchInput=off
  Gain : Gain  Gain=2*pi  SaturateOnIntegerOverflow=on
  Integrator : Integrator
  Mux : Mux  Inputs=2
  Mux1 : Mux  Inputs=3
  Mux2 : Mux  Inputs=3
  capcom : Subsystem
  dead_time_A : Subsystem
  duty_A1 : Fcn  Expr=0.5*2/sqrt(3)*u(1)*(sin(u(2))+(sin(3*u(2))/6)*(third==1))
  duty_A2 : Fcn  Expr=0.5*2/sqrt(3)*u(1)*(sin(u(2)-2*pi/3)+(sin(3*u(2))/6)*(third==1))
  duty_A3 : Fcn  Expr=0.5*2/sqrt(3)*u(1)*(sin(u(2)+2*pi/3)+(sin(3*u(2))/6)*(third==1))
  ma : Fcn  Expr=sqrt(3)/2*sqrt(u(1)^2+u(3)^2)/u(2)
  pulse dropping : Subsystem
  Sw_ABC : Outport
  wires:
  vq_ref/1 -> Mux2/3  "vqref"
  Vdc/1 -> Mux2/2  "vdc"
  vd_ref/1 -> Mux2/1  "vdref"
  ma/1 -> Mux/1
  Mux2/1 -> ma/1
  duty_A3/1 -> Mux1/3
  duty_A2/1 -> Mux1/2
  duty_A1/1 -> Mux1/1
  Gain/1 -> Integrator/1
  Integrator/1 -> Mux/2
  Mux/1 -> duty_A3/1, duty_A2/1, duty_A1/1
  freq/1 -> Gain/1
  capcom/1(S_ABC) -> dead_time_A/1(pwm_A)
  Mux1/1 -> pulse dropping/1(duty_ABC)
  pulse dropping/1(duty_abc) -> capcom/1(duty_abc)
  dead_time_A/1(S_A) -> Sw_ABC/1

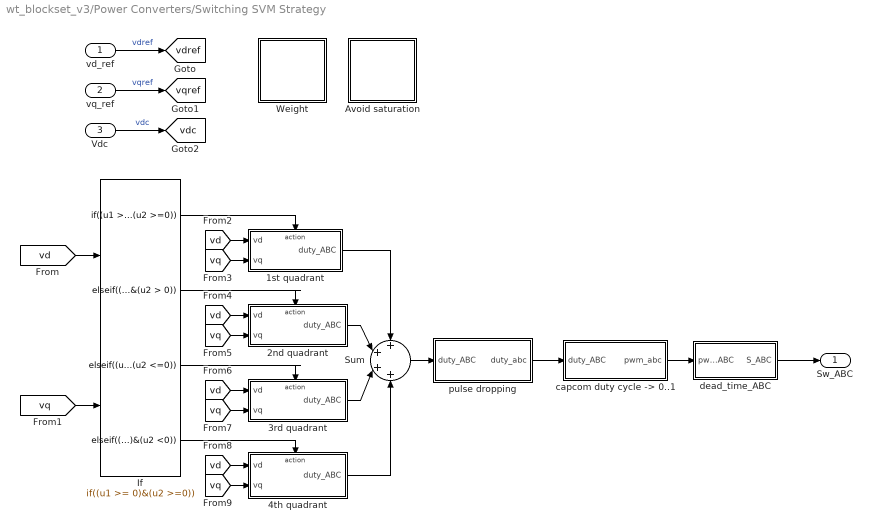
== system wt_blockset_v3/Power Converters/Switching SVM Strategy ==
  vd_ref : Inport  Port=1  LatchInput=off
  vq_ref : Inport  Port=2  LatchInput=off
  Vdc : Inport  Port=3  LatchInput=off
  1st quadrant : Subsystem  TreatAsAtomicUnit=on
  2nd quadrant : Subsystem  TreatAsAtomicUnit=on
  3rd quadrant : Subsystem  TreatAsAtomicUnit=on
  4th quadrant : Subsystem  TreatAsAtomicUnit=on
  "Avoid saturation " : Subsystem
      mask Display: disp('Avoid\nSaturation')
  If : If  NumInputs=2  IfExpression=(u1 >= 0)&(u2 >=0)  ElseIfExpressions=(u1 < 0)&(u2 > 0), (u1 < 0)&(u2 <=0), (u1 >= 0)&(u2 <0)  ShowElse=off
  Sum : Sum  Inputs=++++  SaturateOnIntegerOverflow=on
  Weight : Subsystem
      mask Type: Avoid saturation
      mask Display: disp('Weight')
  "capcom duty cycle -> 0..1" : Subsystem
  dead_time_ABC : Subsystem
  pulse dropping : Subsystem
  Sw_ABC : Outport
  tag scope: vdc=global, vdref=global, vqref=global
  wires:
  vd_ref/1 -> [vdref]  "vdref"
  vq_ref/1 -> [vqref]  "vqref"
  Vdc/1 -> [vdc]  "vdc"
  [vd] -> If/1
  [vq] -> If/2
  If/1 -> 1st quadrant/Action
  [vd] -> 1st quadrant/1(vd)
  [vq] -> 1st quadrant/2(vq)
  [vd] -> 2nd quadrant/1(vd)
  [vq] -> 2nd quadrant/2(vq)
  If/2 -> 2nd quadrant/Action
  [vd] -> 3rd quadrant/1(vd)
  [vq] -> 3rd quadrant/2(vq)
  If/3 -> 3rd quadrant/Action
  [vd] -> 4th quadrant/1(vd)
  [vq] -> 4th quadrant/2(vq)
  If/4 -> 4th quadrant/Action
  1st quadrant/1(duty_ABC) -> Sum/1
  2nd quadrant/1(duty_ABC) -> Sum/2
  4th quadrant/1(duty_ABC) -> Sum/4
  3rd quadrant/1(duty_ABC) -> Sum/3
  dead_time_ABC/1(S_ABC) -> Sw_ABC/1
  "capcom duty cycle -> 0..1"/1(pwm_abc) -> dead_time_ABC/1(pwm_ABC)
  Sum/1 -> pulse dropping/1(duty_ABC)
  pulse dropping/1(duty_abc) -> "capcom duty cycle -> 0..1"/1(duty_ABC)

== system wt_blockset_v3/Power Converters/Switching SVM Strategy C_Sfun ==
  vd_ref : Inport  Port=1  LatchInput=off
  vq_ref : Inport  Port=2  LatchInput=off
  Vdc : Inport  Port=3  LatchInput=off
  Mux : Mux  Inputs=3
  SVM : S-Function  FunctionName=space_vector_mod_sat
  "capcom duty cycle -> 0..1" : Subsystem
  dead_time_A : Subsystem
  pulse dropping : Subsystem
  Sw_ABC : Outport
  wires:
  SVM/1 -> pulse dropping/1(duty_ABC)
  Vdc/1 -> Mux/3
  vq_ref/1 -> Mux/2
  vd_ref/1 -> Mux/1
  Mux/1 -> SVM/1
  "capcom duty cycle -> 0..1"/1(pwm_abc) -> dead_time_A/1(pwm_A)
  dead_time_A/1(S_A) -> Sw_ABC/1
  pulse dropping/1(duty_abc) -> "capcom duty cycle -> 0..1"/1(duty_ABC)

== system wt_blockset_v3/Power Converters/Voltage Source Converter ==
  note: DC-link voltage
  note: Commutation functions
  note: Output voltage
  S_ABC : Inport  Port=1  LatchInput=off
  Vdc : Inport  Port=2  LatchInput=off
  i_ph : Inport  Port=3  LatchInput=off
  DC_link current : Fcn  Expr=u(1)+u(2)+u(3)
  Matrix Gain : Gain  Gain=[2/3 -1/3 -1/3;-1/3 2/3 -1/3;-1/3 -1/3 2/3]  Multiplication=Matrix(u*K)  SaturateOnIntegerOverflow=on
  Product : Product  SaturateOnIntegerOverflow=on  InputSameDT=on
  Product1 : Product  SaturateOnIntegerOverflow=on  InputSameDT=on
  Idc : Outport
  v_ph : Outport  Port=2
  wires:
  Product1/1 -> v_ph/1
  Vdc/1 -> Product1/2
  Matrix Gain/1 -> Product1/1
  S_ABC/1 -> Product/2, Matrix Gain/1
  DC_link current/1 -> Idc/1
  Product/1 -> DC_link current/1
  i_ph/1 -> Product/1

== system wt_blockset_v3/Transformations/ABC->Mag&Phase ==
  ABC : Inport  Port=1  LatchInput=off
  Complex to Magnitude-Angle : ComplexToMagnitudeAngle
  Constant : Constant  Value=j*2*pi/3
  Constant1 : Constant  Value=-j*2*pi/3
  Constant3 : Constant  Value=j*0
  Demux : Demux  Outputs=3
  Gain : Gain  Gain=180/pi  SaturateOnIntegerOverflow=on
  Gain1 : Gain  Gain=2/sqrt(2)/3  SaturateOnIntegerOverflow=on
  Gain3 : Gain  Gain=1/3  SaturateOnIntegerOverflow=on
  Math Function : Math  SaturateOnIntegerOverflow=on
  Math Function1 : Math  SaturateOnIntegerOverflow=on
  Math Function2 : Math  SaturateOnIntegerOverflow=on
  Product1 : Product  SaturateOnIntegerOverflow=on  InputSameDT=on
  Product2 : Product  SaturateOnIntegerOverflow=on  InputSameDT=on
  Product4 : Product  SaturateOnIntegerOverflow=on  InputSameDT=on
  Sum : Sum  Inputs=+++  SaturateOnIntegerOverflow=on  InputSameDT=on
  Sum1 : Sum  Inputs=+++  SaturateOnIntegerOverflow=on  InputSameDT=on
  RMS : Outport
  phase : Outport  Port=2
  zero : Outport  Port=3
  wires:
  Constant/1 -> Math Function/1
  Demux/2 -> Product1/1, Sum1/2
  Math Function/1 -> Product1/2
  Constant1/1 -> Math Function1/1
  Demux/3 -> Product2/1, Sum1/3
  Math Function1/1 -> Product2/2
  Product2/1 -> Sum/3
  Product1/1 -> Sum/2
  Complex to Magnitude-Angle/2 -> Gain/1
  Complex to Magnitude-Angle/1 -> Gain1/1
  Gain1/1 -> RMS/1
  ABC/1 -> Demux/1
  Gain/1 -> phase/1
  Product4/1 -> Sum/1
  Demux/1 -> Product4/1, Sum1/1
  Constant3/1 -> Math Function2/1
  Math Function2/1 -> Product4/2
  Sum/1 -> Complex to Magnitude-Angle/1
  Sum1/1 -> Gain3/1
  Gain3/1 -> zero/1

== system wt_blockset_v3/Transformations/DQ -> Complex ==
  A_dq : Inport  Port=1  LatchInput=off
  Gain : Gain  Gain=-1  SaturateOnIntegerOverflow=on
  Real-Imag to Complex : RealImagToComplex
  Selector : Selector  Elements=[2]  InputPortWidth=2
  Selector1 : Selector  Elements=[1]  InputPortWidth=2
  A_cmpl : Outport
  wires:
  Real-Imag to Complex/1 -> A_cmpl/1
  A_dq/1 -> Selector/1, Selector1/1
  Selector/1 -> Real-Imag to Complex/1
  Selector1/1 -> Gain/1
  Gain/1 -> Real-Imag to Complex/2

== system wt_blockset_v3/Transformations/abc -> dq0 ==
  ABC : Inport  Port=1  LatchInput=off
  theta : Inport  Port=2  LatchInput=off
  Mux : Mux  Inputs=[3 1]
  Mux1 : Mux  Inputs=3
  v0 : Fcn  Expr=(u(1)+u(2)+u(3))/3
  vd : Fcn  Expr=2*(u[1]*cos(u[4])+u[2]*cos(u[4]-2*pi/3)+u[3]*cos(u[4]+2*pi/3))/3
  vq : Fcn  Expr=-2*(u[1]*sin(u[4])+u[2]*sin(u[4]-2*pi/3)+u[3]*sin(u[4]+2*pi/3))/3
  DQO : Outport  InitialOutput=0
  wires:
  theta/1 -> Mux/2
  Mux1/1 -> DQO/1
  Mux/1 -> vd/1, vq/1, v0/1
  ABC/1 -> Mux/1
  vd/1 -> Mux1/1
  vq/1 -> Mux1/2
  v0/1 -> Mux1/3

== system wt_blockset_v3/Transformations/dq0 -> abc ==
  DQO : Inport  Port=1  LatchInput=off
  theta : Inport  Port=2  LatchInput=off
  Mux : Mux  Inputs=[3 1]
  Mux1 : Mux  Inputs=3
  va : Fcn  Expr=u[1]*cos(u[4])-u[2]*sin(u[4])+u(3)
  vb : Fcn  Expr=u[1]*cos(u[4]-2*pi/3)-u[2]*sin(u[4]-2*pi/3)+u(3)
  vc : Fcn  Expr=u[1]*cos(u[4]+2*pi/3)-u[2]*sin(u[4]+2*pi/3)+u(3)
  ABC : Outport  InitialOutput=0
  wires:
  theta/1 -> Mux/2
  Mux1/1 -> ABC/1
  vc/1 -> Mux1/3
  vb/1 -> Mux1/2
  va/1 -> Mux1/1
  DQO/1 -> Mux/1
  Mux/1 -> va/1, vb/1, vc/1

== system wt_blockset_v3/Transformations/phase -> line currents ==
  i_phase : Inport  Port=1  LatchInput=off
  phase ->line currents : Gain  Gain=[1 0 -1;-1 1 0;0 -1 1]  Multiplication=Matrix(K*u)  SaturateOnIntegerOverflow=on
  i_line : Outport
  wires:
  i_phase/1 -> phase ->line currents/1
  phase ->line currents/1 -> i_line/1

== system wt_blockset_v3/Transformations/phase->line voltages ==
  v_phase : Inport  Port=1  LatchInput=off
  phase ->line voltages : Gain  Gain=[1 -1 0; 0 1 -1; -1 0 1]  Multiplication=Matrix(K*u)  SaturateOnIntegerOverflow=on
  v_line : Outport
  wires:
  phase ->line voltages/1 -> v_line/1
  v_phase/1 -> phase ->line voltages/1

== system wt_blockset_v3/Control/Active Stall Controller /MAF_wind ==
  In : Inport  Port=1  LatchInput=off
  Constant : Constant  Value=init
  Gain : Gain  Gain=1/Tav  SaturateOnIntegerOverflow=on
  Integrator : Integrator
  Sum : Sum  Inputs=|+-  SaturateOnIntegerOverflow=on
  Sum1 : Sum  Inputs=|++  SaturateOnIntegerOverflow=on
  Transport Delay : TransportDelay  DelayTime=Tav  InitialInput=init  BufferSize=6144  TransDelayFeedthrough=on
  Out : Outport
  wires:
  Sum1/1 -> Out/1
  Constant/1 -> Sum1/2
  Gain/1 -> Sum1/1
  Integrator/1 -> Gain/1
  Sum/1 -> Integrator/1
  Transport Delay/1 -> Sum/2
  In/1 -> Sum/1, Transport Delay/1

== system wt_blockset_v3/Control/Active Stall Controller /MAF_wind1 ==
  In : Inport  Port=1  LatchInput=off
  Constant : Constant  Value=init
  Gain : Gain  Gain=1/Tav  SaturateOnIntegerOverflow=on
  Integrator : Integrator
  Sum : Sum  Inputs=|+-  SaturateOnIntegerOverflow=on
  Sum1 : Sum  Inputs=|++  SaturateOnIntegerOverflow=on
  Transport Delay : TransportDelay  DelayTime=Tav  InitialInput=init  BufferSize=6144  TransDelayFeedthrough=on
  Out : Outport
  wires:
  Sum1/1 -> Out/1
  Constant/1 -> Sum1/2
  Gain/1 -> Sum1/1
  Integrator/1 -> Gain/1
  Sum/1 -> Integrator/1
  Transport Delay/1 -> Sum/2
  In/1 -> Sum/1, Transport Delay/1

== system wt_blockset_v3/Control/Active Stall Controller /Pitch System ==
  In : Inport  Port=1  LatchInput=off
  Rate Limiter : RateLimiter  RisingSlewLimit=8  FallingSlewLimit=-8
  Saturation1 : Saturate  UpperLimit=2  LowerLimit=-10
  Out : Outport
  wires:
  Rate Limiter/1 -> Saturation1/1
  In/1 -> Rate Limiter/1
  Saturation1/1 -> Out/1

== system wt_blockset_v3/Control/Active Stall Controller /Power Controller ==
  error : Inport  Port=1  LatchInput=off
  aw : Inport  Orientation=left  Port=2  LatchInput=off
  1/T : Gain  Gain=Ti  SaturateOnIntegerOverflow=on
  Integrator : Integrator
  P1 : Gain  Gain=K  SaturateOnIntegerOverflow=on
  P2 : Gain  Orientation=left  Gain=ka  SaturateOnIntegerOverflow=on
  Saturation : Saturate  UpperLimit=+2  LowerLimit=-10
  Sum1 : Sum  Inputs=|+-  SaturateOnIntegerOverflow=on  InputSameDT=on
  Sum2 : Sum  Inputs=++|  SaturateOnIntegerOverflow=on  InputSameDT=on
  Sum4 : Sum  Orientation=left  Inputs=+-|  SaturateOnIntegerOverflow=on  InputSameDT=on
  pitch : Outport
  wires:
  1/T/1 -> Integrator/1
  Integrator/1 -> Sum2/2
  Sum1/1 -> 1/T/1
  Sum2/1 -> Sum4/1, Saturation/1
  Sum4/1 -> P2/1
  P1/1 -> Sum2/1
  P2/1 -> Sum1/2
  aw/1 -> Sum4/2
  error/1 -> P1/1, Sum1/1
  Saturation/1 -> pitch/1  "pitch PI"

== system wt_blockset_v3/Control/Active Stall Controller /Sample and Hold ==
  In : Inport  Port=1  LatchInput=off
  Trigger : TriggerPort  ZeroCross=off
  " " : Outport  InitialOutput=initCond
  wires:
  In/1 -> " "/1

== system wt_blockset_v3/Control/Active Stall Controller /control ==
  av_wind : Inport  Orientation=down  Port=1  LatchInput=off
  error : Inport  Port=2  LatchInput=off
  Data Type Conversion1 : DataTypeConversion  SaturateOnIntegerOverflow=on  RndMeth=Zero
  Logical Operator1 : Logic  AllPortsSameDT=off
  meas1 : Constant  Value=2000
  meas4 : Constant  Value=rated_wind
  overpower  detection : RelationalOperator  Operator=>
  overpower  detection3 : RelationalOperator  Operator=<
  cs : Outport
  wires:
  meas1/1 -> overpower  detection/1
  meas4/1 -> overpower  detection3/2
  Logical Operator1/1 -> Data Type Conversion1/1  "cs1"
  overpower  detection3/1 -> Logical Operator1/1
  overpower  detection/1 -> Logical Operator1/2
  av_wind/1 -> overpower  detection3/1
  error/1 -> overpower  detection/2
  Data Type Conversion1/1 -> cs/1

== system wt_blockset_v3/Control/Active Stall Controller /trigger ==
  overpower : Inport  Port=1  LatchInput=off
  Fast : DiscretePulseGenerator  PulseType=Time based  Period=5  PulseWidth=10
  Slow : DiscretePulseGenerator  PulseType=Time based  Period=60  PulseWidth=10
  Switch1 : Switch  Threshold=0.5  SaturateOnIntegerOverflow=on
  trigger : Outport
  wires:
  Slow/1 -> Switch1/3
  Fast/1 -> Switch1/1
  overpower/1 -> Switch1/2
  Switch1/1 -> trigger/1

== system wt_blockset_v3/Control/Control P&Q  2 MW DFIG/PI regulator1 ==
  ref : Inport  Port=1  LatchInput=off
  meas : Inport  Port=2  LatchInput=off
  1/T : Gain  Gain=1/Ti  SaturateOnIntegerOverflow=on
  Integrator : Integrator  InitialCondition=init_cond
  P1 : Gain  Gain=K  SaturateOnIntegerOverflow=on
  P2 : Gain  Orientation=left  Gain=ka  SaturateOnIntegerOverflow=on
  Saturation : Saturate  UpperLimit=maxim  LowerLimit=-maxim
  Sum1 : Sum  Inputs=|+-  SaturateOnIntegerOverflow=on  InputSameDT=on
  Sum2 : Sum  Inputs=++|  SaturateOnIntegerOverflow=on  InputSameDT=on
  Sum3 : Sum  Inputs=|+-  SaturateOnIntegerOverflow=on  InputSameDT=on
  Sum4 : Sum  Orientation=left  Inputs=+-|  SaturateOnIntegerOverflow=on  InputSameDT=on
  out : Outport  InitialOutput=0
  wires:
  Saturation/1 -> Sum4/2, out/1
  Sum2/1 -> Saturation/1, Sum4/1
  meas/1 -> Sum3/2
  P1/1 -> Sum2/1, Sum1/1
  ref/1 -> Sum3/1
  Sum3/1 -> P1/1
  1/T/1 -> Integrator/1
  Integrator/1 -> Sum2/2
  Sum1/1 -> 1/T/1
  Sum4/1 -> P2/1
  P2/1 -> Sum1/2

== system wt_blockset_v3/Control/Control P&Q  2 MW DFIG/PI regulator2 ==
  ref : Inport  Port=1  LatchInput=off
  meas : Inport  Port=2  LatchInput=off
  1/T : Gain  Gain=1/Ti  SaturateOnIntegerOverflow=on
  Integrator : Integrator  InitialCondition=init_cond
  P1 : Gain  Gain=K  SaturateOnIntegerOverflow=on
  P2 : Gain  Orientation=left  Gain=ka  SaturateOnIntegerOverflow=on
  Saturation : Saturate  UpperLimit=maxim  LowerLimit=-maxim
  Sum1 : Sum  Inputs=|+-  SaturateOnIntegerOverflow=on  InputSameDT=on
  Sum2 : Sum  Inputs=++|  SaturateOnIntegerOverflow=on  InputSameDT=on
  Sum3 : Sum  Inputs=|+-  SaturateOnIntegerOverflow=on  InputSameDT=on
  Sum4 : Sum  Orientation=left  Inputs=+-|  SaturateOnIntegerOverflow=on  InputSameDT=on
  out : Outport  InitialOutput=0
  wires:
  Saturation/1 -> Sum4/2, out/1
  Sum2/1 -> Saturation/1, Sum4/1
  meas/1 -> Sum3/2
  P1/1 -> Sum2/1, Sum1/1
  ref/1 -> Sum3/1
  Sum3/1 -> P1/1
  1/T/1 -> Integrator/1
  Integrator/1 -> Sum2/2
  Sum1/1 -> 1/T/1
  Sum4/1 -> P2/1
  P2/1 -> Sum1/2
